simulink model "SlidingModeAdaptiveControl_HW"  (R2019a)
settings: Solver=VariableStepAuto  StartTime=0.0  StopTime=10.0  RelTol=1e-3
InitFcn:
  | ini_file_HW
values from neighbouring files (symbols this model uses):
  gamma = 3    [ini_file_HW.m]
  lambda1 = 10    [ini_file_HW.m]
  lambda2 = 25    [ini_file_HW.m]
settings Model: Creator=0629w  LastModifiedBy=0629w

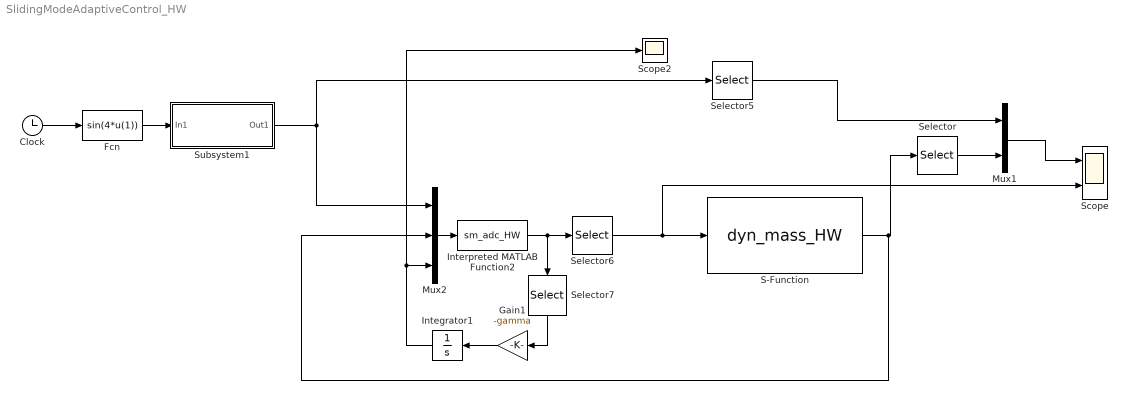
== system SlidingModeAdaptiveControl_HW ==
  Clock : Clock
  Fcn : Fcn  Expr=sin(4*u(1))
  Gain1 : Gain  Gain=-gamma
  Integrator1 : Integrator
  Interpreted MATLAB Function2 : MATLABFcn  MATLABFcn=sm_adc_HW  OutputDimensions=2
  Mux1 : Mux  Inputs=2
  Mux2 : Mux  Inputs=3
  S-Function : S-Function  FunctionName=dyn_mass_HW  SFunctionDeploymentMode=off  EnableBusSupport=off
  Scope : Scope  NumInputPorts=2
  Scope2 : Scope
  Selector : Selector  InputPortWidth=2  IndexOptions=Index vector (dialog)  Indices=[1]  OutputSizes=1
  Selector5 : Selector  InputPortWidth=3  IndexOptions=Index vector (dialog)  Indices=[1]  OutputSizes=1
  Selector6 : Selector  InputPortWidth=2  IndexOptions=Index vector (dialog)  Indices=[1]  OutputSizes=1
  Selector7 : Selector  IndexMode=Zero-based  InputPortWidth=2  IndexOptions=Index vector (dialog)  Indices=[1]  OutputSizes=1
  Subsystem1 : Subsystem
  wires:
  Clock/1 -> Fcn/1
  S-Function/1 -> Mux2/2, Selector/1
  Mux1/1 -> Scope/1
  Selector/1 -> Mux1/2
  Selector5/1 -> Mux1/1
  Gain1/1 -> Integrator1/1
  Mux2/1 -> Interpreted MATLAB Function2/1
  Selector7/1 -> Gain1/1
  Interpreted MATLAB Function2/1 -> Selector6/1, Selector7/1
  Integrator1/1 -> Scope2/1, Mux2/3
  Selector6/1 -> Scope/2, S-Function/1
  Fcn/1 -> Subsystem1/1(In1)
  Subsystem1/1(Out1) -> Selector5/1, Mux2/1

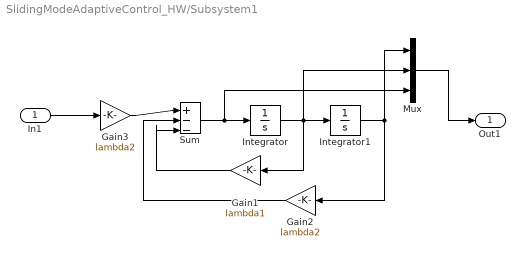
== system SlidingModeAdaptiveControl_HW/Subsystem1 ==
  In1 : Inport
  Gain1 : Gain  Gain=lambda1
  Gain2 : Gain  Gain=lambda2
  Gain3 : Gain  Gain=lambda2
  Integrator : Integrator
  Integrator1 : Integrator
  Mux : Mux  Inputs=3
  Sum : Sum  Inputs=|+--
  Out1 : Outport
  wires:
  In1/1 -> Gain3/1
  Gain3/1 -> Sum/1
  Sum/1 -> Mux/3, Integrator/1
  Integrator/1 -> Gain1/1, Mux/2, Integrator1/1
  Integrator1/1 -> Gain2/1, Mux/1
  Gain1/1 -> Sum/3
  Gain2/1 -> Sum/2
  Mux/1 -> Out1/1
